simulink model "sedemo_rate_based_proc"  (Simulink 7.5)
settings: Solver=VariableStepDiscrete  StartTime=0.0  StopTime=86  MaxStep=Inf  RelTol=1e-3
undefined symbols (not defined in the file or in its folder): des_subsystemblock, des_subsysteminport, des_subsystemoutport, des_subsystemsupportblock
libraries: simeventstiming1 x7, simeventstranslate1 x7, simeventssink1 x5, simeventsattributes2 x5, simeventsgenerators1 x4, simeventsgates1 x3, simeventsrouting1 x3, simeventsserver1 x3, simeventsqueue1 x1, simeventsinfo x1
settings Model: Creator=The MathWorks Inc.
settings SolverCC: InsertRTBMode=Auto
settings OptimizationCC: InitFltsAndDblsToZero=on
settings DebuggingCC: SolverPrmCheckMsg=none  StrictBusMsg=Warning
settings SimEventsCC: propMaxDesBlkSimulEvents=10000  propDiagAttribOutput=0  propDiagFcnCallOutput=0  propDiagStatOutput=0  propDiagChangeAttrib=0  propRNGIdenticalSeeds=0

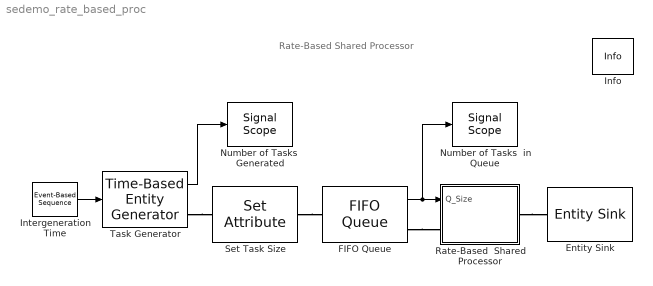
== system sedemo_rate_based_proc ==
  note: Rate-Based Shared Processor
  Entity Sink : simeventssink1/Entity Sink  Priority=1  SystemSampleTime=-1  AvailableForArrivals=on  StatNumberArrived=Off
  FIFO Queue : simeventsqueue1/FIFO Queue  Priority=1  SystemSampleTime=-1  Capacity=10  EnableTOPort=off  StatNumberDeparted=Off  StatNumberInBlock=On  StatPendingEntity=Off  StatAverageWait=Off  StatAverageQueueLength=Off  StatNumberTimedout=Off
  Info : simeventsinfo/Info  SystemSampleTime=-1
  Intergeneration Time : simeventsgenerators1/Signal Generators/Event-Based Sequence  SystemSampleTime=-1  VectorOutputValues=rand(1,85)*2.4  FormOutputOpt=Cyclic repetition  IsProcessed=on  isConnected=1
  Number of Tasks  Generated : simeventssink1/Signal Scope  Priority=1  SystemSampleTime=-1  PlotType=Stair  InputType=Signal  NumInputs=1  AttributeNameY=Count  XInputOptionSignal=Event time  XInputOptionEntity=Event time  AttributeNameX=Count  EnableEntityOutport=on  XMin=0  XMax=100  XLimitExceededOption=Stretch axis limits  YLimitExceededOption=Stretch axis limits  AxisGrid=on  AxisLegend=off  LineDisables=""  LineColors=b  LineStyles=-  LineMarkers=None  OpenScopeAtSimStart=on  Title=Number of Tasks Generated  YLabel=Number of Tasks  XLabel=Time  FigurePosition=[116 516 360 184]  AxisZoom=off  DataStoreOption=Limited  DataPointsLimit=10000  StatNumberArrived=Off  ShowCountPlotted=off  ShowToolbar=off
      settings: YMin=0  YMax=100
  Number of Tasks  in Queue : simeventssink1/Signal Scope  Priority=1  SystemSampleTime=-1  PlotType=Stair  InputType=Signal  NumInputs=1  AttributeNameY=Count  XInputOptionSignal=Event time  XInputOptionEntity=Event time  AttributeNameX=Count  EnableEntityOutport=on  XMin=0  XMax=100  XLimitExceededOption=Stretch axis limits  YLimitExceededOption=Stretch axis limits  AxisGrid=on  AxisLegend=off  LineDisables=""  LineColors="1  0  1"  LineStyles=-  LineMarkers=None  OpenScopeAtSimStart=on  Title=Number of Tasks Waiting for Service  YLabel=Number of Tasks  XLabel=Time  FigurePosition=[483 516 360 184]  AxisZoom=off  DataStoreOption=Limited  DataPointsLimit=10000  StatNumberArrived=Off  ShowCountPlotted=off  ShowToolbar=off
      settings: YMin=0  YMax=4
  Rate-Based  Shared Processor : Subsystem
  Set Task Size : simeventsattributes2/Set Attribute  Priority=1  DialogController=des_ddg_create  DialogControllerArgs=DataTag62  SystemSampleTime=-1  AttributeFrom=Dialog  AttributeName=ResidualWork  AttributeTreatAsVector=1  AttributeValue=1  AttributeCreate=on  StatNumberDeparted=Off  EvaluatedAttributeValue={1}
  Task Generator : simeventsgenerators1/Entity Generators/Time-Based Entity Generator  Priority=1  DialogController=des_ddg_create  DialogControllerArgs=DataTag64  SystemSampleTime=-1  GenerateEntitiesUpon=Intergeneration time from port t  Distribution=Exponential  Minimum=0  Maximum=1  Mean=2  InitialSeed=9675678  Period=1  PriorityEntityGeneration=300  GenerateEntityAtSimulationStart=on  ResponseWhenBlocked=Pause generation  ResponseWhenUnblocked=Immediate restart  EntityType=Blank  StatNumberDeparted=On  StatPendingEntity=Off  StatAverageIntergenerationTime=Off
  wires:
  FIFO Queue/1 -> Rate-Based  Shared Processor/1(Q_Size), Number of Tasks  in Queue/1
  Intergeneration Time/1 -> Task Generator/1
  Task Generator/1 -> Number of Tasks  Generated/1
  connections:
  Task Generator/RConn1 -- Set Task Size/LConn1
  FIFO Queue/RConn1 -- Rate-Based  Shared Processor/LConn1
  Rate-Based  Shared Processor/RConn1 -- Entity Sink/LConn1
  Set Task Size/RConn1 -- FIFO Queue/LConn1

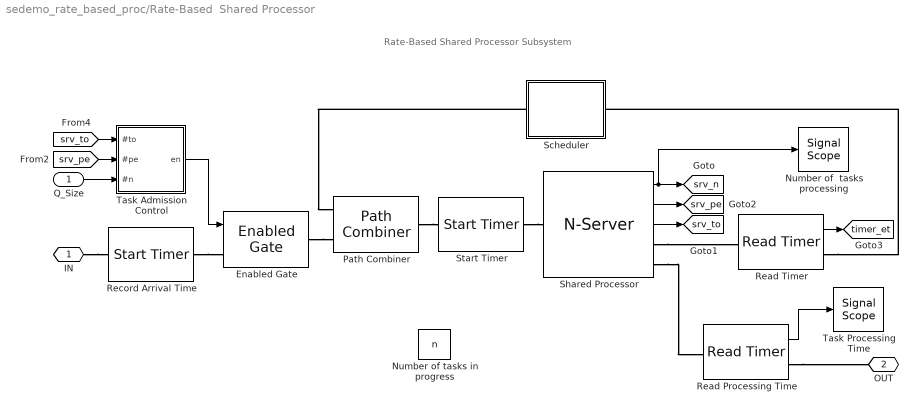
== system sedemo_rate_based_proc/Rate-Based  Shared Processor ==
  note: Rate-Based Shared Processor Subsystem
  Q_Size : Inport  OutDataType=sfix(16)  OutScaling=2^0
  Enabled Gate : simeventsgates1/Enabled Gate  Priority=1  SystemSampleTime=-1  SpecifyEventPriority=off  PriorityGateEnableOpenClose=2000  StatNumberDeparted=Off
  Number of  tasks processing : simeventssink1/Signal Scope  Priority=1  SystemSampleTime=-1  PlotType=Stair  InputType=Signal  NumInputs=1  AttributeNameY=Count  XInputOptionSignal=Event time  XInputOptionEntity=Event time  AttributeNameX=Count  EnableEntityOutport=on  XMin=0  XMax=100  XLimitExceededOption=Stretch axis limits  YLimitExceededOption=Stretch axis limits  AxisGrid=on  AxisLegend=off  LineDisables=""  LineColors="1  0  0"  LineStyles=-  LineMarkers=None  OpenScopeAtSimStart=on  Title=Number of Tasks Being Processed  YLabel=Number of Tasks  XLabel=Time  FigurePosition=[116 283 360 185]  AxisZoom=off  DataStoreOption=Limited  DataPointsLimit=10000  StatNumberArrived=Off  ShowCountPlotted=off  ShowToolbar=off
      settings: YMin=0  YMax=6
  Number of tasks in progress : DataStoreMemory  DataStoreName=n  OutDataType=sfix(16)  OutScaling=2^0
  Path Combiner : simeventsrouting1/Path Combiner  Priority=1  SystemSampleTime=-1  NumberInputPorts=2  InputPortPrecedence=IN1 port  InitialSeed=45675  SpecifyEventPriority=off  PriorityPathCombinerPortPrecedenceSelection=4100  StatNumberDeparted=Off  StatLastArrivalPort=Off  EvaluatedNumPorts=2
  Read Processing Time : simeventstiming1/Read Timer  Priority=0  SystemSampleTime=-1  TimerTag=ProcessingTime  TimerModeOption=Error  TimerStop=off  StatNumberDeparted=Off  StatTimerNumberDeparted=Off  StatTimeElapsed=On  StatAverageTimeElapsed=Off
  Read Timer : simeventstiming1/Read Timer  Priority=0  SystemSampleTime=-1  TimerTag=ServiceTime  TimerModeOption=Error  TimerStop=off  StatNumberDeparted=Off  StatTimerNumberDeparted=Off  StatTimeElapsed=On  StatAverageTimeElapsed=Off
  Record Arrival Time : simeventstiming1/Start Timer  Priority=0  SystemSampleTime=-1  TimerTag=ProcessingTime  TimerStartedOption=Warn and continue  StatNumberDeparted=Off
  Scheduler : Subsystem
  Shared Processor : simeventsserver1/N-Server  Priority=1  SystemSampleTime=-1  NumberOfServers=5  ServiceTimeFrom=Dialog  ServiceTime=0  AttributeName=ServiceTime  PriorityServiceCompletion=700  EnableTOPort=on  StatNumberDeparted=Off  StatNumberInBlock=On  StatPendingEntity=Off  StatNumberPending=On  StatAverageWait=Off  StatUtilization=Off  StatNumberTimedout=On
  Start Timer : simeventstiming1/Start Timer  Priority=0  SystemSampleTime=-1  TimerTag=ServiceTime  TimerStartedOption=Restart  StatNumberDeparted=Off
  Task Admission Control : Subsystem  LoadFcn=des_subsystemblock(gcb, 'load');  InitFcn=des_subsystemblock(gcb, 'init');  StartFcn=des_subsystemblock(gcb, 'start');  StopFcn=des_subsystemblock(gcb, 'stop');
      settings: CopyFcn=des_subsystemblock(gcb, 'copy');  DeleteFcn=des_subsystemblock(gcb, 'delete');  UndoDeleteFcn=des_subsystemblock(gcb, 'undodelete');  ModelCloseFcn=des_subsystemblock(gcb, 'modelclose');  PreSaveFcn=des_subsystemblock(gcb, 'presave');  NameChangeFcn=des_subsystemblock(gcb, 'namechange');  ParentCloseFcn=des_subsystemblock(gcb, 'parentclose');  ErrorFcn=des_subsystemerror
  Task Processing Time : simeventssink1/Signal Scope  Priority=1  SystemSampleTime=-1  PlotType=Stem  InputType=Signal  NumInputs=1  AttributeNameY=Count  XInputOptionSignal=Event time  XInputOptionEntity=Event time  AttributeNameX=Count  EnableEntityOutport=on  XMin=0  XMax=100  XLimitExceededOption=Stretch axis limits  YLimitExceededOption=Stretch axis limits  AxisGrid=on  AxisLegend=off  LineDisables=""  LineColors="0  0  1"  LineStyles=-  LineMarkers=diamond  OpenScopeAtSimStart=on  Title=Task Processing Time  YLabel=Processing Time  XLabel=Departure Time  FigurePosition=[483 283 360 185]  AxisZoom=off  DataStoreOption=Limited  DataPointsLimit=10000  StatNumberArrived=Off  ShowCountPlotted=off  ShowToolbar=off
      settings: YMin=0  YMax=6
  IN : PMIOPort  Port=1  Side=Left
  OUT : PMIOPort  Port=2  Side=Right
  tag scope: srv_n=global, srv_pe=global, srv_to=global, timer_et=global
  wires:
  Read Timer/1 -> [timer_et]
  Shared Processor/1 -> [srv_n], Number of  tasks processing/1
  Shared Processor/2 -> [srv_pe]
  Shared Processor/3 -> [srv_to]
  Task Admission Control/1(en) -> Enabled Gate/1
  Q_Size/1 -> Task Admission Control/3(#n)
  [srv_pe] -> Task Admission Control/2(#pe)
  [srv_to] -> Task Admission Control/1(#to)
  Read Processing Time/1 -> Task Processing Time/1
  connections:
  Start Timer/RConn1 -- Shared Processor/LConn1
  Shared Processor/RConn1 -- Read Timer/LConn1
  Path Combiner/RConn1 -- Start Timer/LConn1
  Enabled Gate/RConn1 -- Path Combiner/LConn2
  Read Timer/RConn1 -- Scheduler/LConn1
  Scheduler/RConn1 -- Path Combiner/LConn1
  Record Arrival Time/RConn1 -- Enabled Gate/LConn1
  IN/RConn1 -- Record Arrival Time/LConn1
  Shared Processor/RConn2 -- Read Processing Time/LConn1
  Read Processing Time/RConn1 -- OUT/RConn1

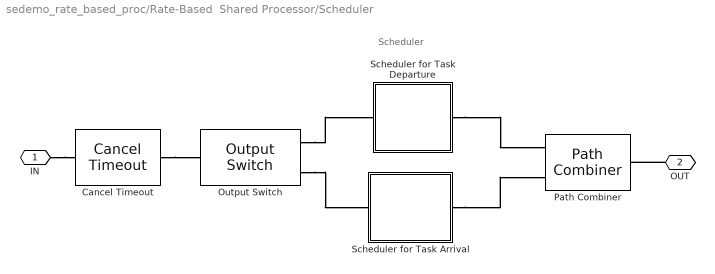
== system sedemo_rate_based_proc/Rate-Based  Shared Processor/Scheduler ==
  note: Scheduler
  Cancel Timeout : simeventstiming1/Cancel Timeout  Priority=0  SystemSampleTime=-1  TimeoutTag=ResidualServiceTime  TimeoutModeOption=Continue  TimeoutCancelledOption=Continue  StatNumberDeparted=Off  StatTimeoutNumberDeparted=Off  StatResidualTimeout=Off  StatAverageResidualTimeout=Off
  Output Switch : simeventsrouting1/Output Switch  Priority=1  SystemSampleTime=-1  NumberOutputPorts=2  SwitchingCriterion=First port that is not blocked  InitialSeed=34567  AttributeName=Attribute1  InitialConditionsOpt=off  InitialConditions=1  EntityBufferOpt=off  SpecifyEventPriority=off  PriorityOutputSwitchSelectPort=4100  TimeoutPortOpt=off  StatNumberDeparted=Off  StatNumberTimedOut=Off  StatPendingEntity=Off  StatLastDeparturePort=Off  EvaluatedNumPorts=2
  Path Combiner : simeventsrouting1/Path Combiner  Priority=1  SystemSampleTime=-1  NumberInputPorts=2  InputPortPrecedence=IN1 port  InitialSeed=45675  SpecifyEventPriority=off  PriorityPathCombinerPortPrecedenceSelection=4100  StatNumberDeparted=Off  StatLastArrivalPort=Off  EvaluatedNumPorts=2
  Scheduler for Task Arrival : Subsystem
  Scheduler for Task Departure : Subsystem
  IN : PMIOPort  Port=1  Side=Left
  OUT : PMIOPort  Port=2  Side=Right
  connections:
  Cancel Timeout/RConn1 -- Output Switch/LConn1
  Output Switch/RConn1 -- Scheduler for Task Departure/LConn1
  Output Switch/RConn2 -- Scheduler for Task Arrival/LConn1
  Scheduler for Task Departure/RConn1 -- Path Combiner/LConn1
  Scheduler for Task Arrival/RConn1 -- Path Combiner/LConn2
  IN/RConn1 -- Cancel Timeout/LConn1
  OUT/RConn1 -- Path Combiner/RConn1

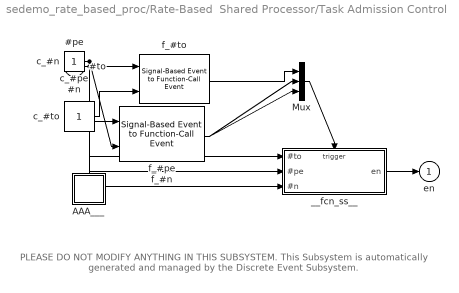
== system sedemo_rate_based_proc/Rate-Based  Shared Processor/Task Admission Control ==
  note: PLEASE DO NOT MODIFY ANYTHING IN THIS SUBSYSTEM.
      | This Subsystem is automatically generated and
      | managed by the Discrete Event Subsystem.
  #to : Inport  DataType=double  OutDataType=sfix(16)  OutScaling=2^0  OutDataTypeStr=double
  #pe : Inport  Port=2  DataType=double  OutDataType=sfix(16)  OutScaling=2^0  OutDataTypeStr=double
  #n : Inport  Port=3  DataType=double  OutDataType=sfix(16)  OutScaling=2^0  OutDataTypeStr=double
  AAA___ : Subsystem  LoadFcn=des_subsystemsupportblock(gcb, 'load');  InitFcn=des_subsystemsupportblock(gcb, 'init');  StartFcn=des_subsystemsupportblock(gcb, 'start');  StopFcn=des_subsystemsupportblock(gcb, 'stop');
      settings: CopyFcn=des_subsystemsupportblock(gcb, 'copy');  DeleteFcn=des_subsystemsupportblock(gcb, 'delete');  UndoDeleteFcn=des_subsystemsupportblock(gcb, 'undodelete');  ModelCloseFcn=des_subsystemsupportblock(gcb, 'modelclose');  PreSaveFcn=des_subsystemsupportblock(gcb, 'presave');  NameChangeFcn=des_subsystemsupportblock(gcb, 'namechange');  OpenFcn=des_subsystemsupportblock(gcb, 'open');  ParentCloseFcn=des_subsystemsupportblock(gcb, 'parentclose');
  Mux : Mux  Inputs=3
  __fcn_ss__ : Subsystem  TreatAsAtomicUnit=on
      settings: PropExecContextOutsideSubsystem=on
  c_#n : Constant  OutDataType=sfix(16)  OutScaling=2^0
  c_#pe : Constant  OutDataType=sfix(16)  OutScaling=2^0
  c_#to : Constant  OutDataType=sfix(16)  OutScaling=2^0
  f_#n : simeventstranslate1/Signal-Based Event to Function-Call Event  Priority=1  SystemSampleTime=-1  GenerateFunctionCallUpon=Change in signal from port vc  SignalEdgeOption=Rising  EnableE1Port=on  EnableF2Port=off  EnableE2Port=off  SpecifyEventPriority=off  PriorityFunctionCall=600  FunctionCallDelayFrom=Dialog  DelayFunctionCall=0  StatNumberF1Calls=Off  StatNumberF2Calls=Off  MaskBlockType=DESS_EVENT_PORT
  f_#pe : simeventstranslate1/Signal-Based Event to Function-Call Event  Priority=1  SystemSampleTime=-1  GenerateFunctionCallUpon=Change in signal from port vc  SignalEdgeOption=Rising  EnableE1Port=on  EnableF2Port=off  EnableE2Port=off  SpecifyEventPriority=off  PriorityFunctionCall=800  FunctionCallDelayFrom=Dialog  DelayFunctionCall=0  StatNumberF1Calls=Off  StatNumberF2Calls=Off  MaskBlockType=DESS_EVENT_PORT
  f_#to : simeventstranslate1/Signal-Based Event to Function-Call Event  Priority=1  SystemSampleTime=-1  GenerateFunctionCallUpon=Change in signal from port vc  SignalEdgeOption=Rising  EnableE1Port=on  EnableF2Port=off  EnableE2Port=off  SpecifyEventPriority=off  PriorityFunctionCall=500  FunctionCallDelayFrom=Dialog  DelayFunctionCall=0  StatNumberF1Calls=Off  StatNumberF2Calls=Off  MaskBlockType=DESS_EVENT_PORT
  en : Outport  OutDataType=sfix(16)  OutScaling=2^0
  wires:
  c_#pe/1 -> f_#pe/2
  f_#pe/1 -> Mux/2
  Mux/1 -> __fcn_ss__/Trigger
  c_#to/1 -> f_#to/2
  f_#to/1 -> Mux/1
  __fcn_ss__/1(en) -> en/1
  f_#n/1 -> Mux/3
  c_#n/1 -> f_#n/2
  #to/1 -> f_#to/1, __fcn_ss__/1(#to)
  #pe/1 -> f_#pe/1, __fcn_ss__/2(#pe)
  #n/1 -> f_#n/1, __fcn_ss__/3(#n)

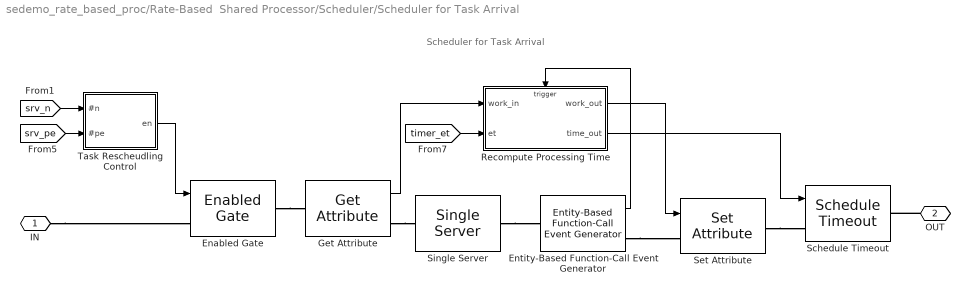
== system sedemo_rate_based_proc/Rate-Based  Shared Processor/Scheduler/Scheduler for Task Arrival ==
  note: Scheduler for Task Arrival
  Enabled Gate : simeventsgates1/Enabled Gate  Priority=1  SystemSampleTime=-1  SpecifyEventPriority=off  PriorityGateEnableOpenClose=2000  StatNumberDeparted=Off
  Entity-Based Function-Call Event Generator : simeventsgenerators1/Event Generators/Entity-Based Function-Call Event Generator  Priority=1  SystemSampleTime=-1  TimingFunctionCallF1=Before entity departure  EnableE1Port=off  EnableF2Port=off  TimingFunctionCallF2=After entity departure  EnableE2Port=off  StatNumberDeparted=Off  StatNumberF1Calls=Off  StatNumberF2Calls=Off  IsInsideAFB=off
  Get Attribute : simeventsattributes2/Get Attribute  Priority=1  DialogController=des_ddg_create  DialogControllerArgs=DataTag16  SystemSampleTime=-1  AttributeName=ResidualWork  AttributeMissing=Error  AttributeDefaultValue=1  AttributeSendTiming=After entity departure  AttributeTreatAsVector=1  StatNumberDeparted=Off  EvaluatedDefaultAttributeValue={[]}
  Recompute Processing Time : Subsystem  TreatAsAtomicUnit=on
      settings: PropExecContextOutsideSubsystem=on
  Schedule Timeout : simeventstiming1/Schedule Timeout  Priority=0  SystemSampleTime=-1  TimeoutTag=ResidualServiceTime  TimeoutIntervalFrom=Signal port ti  TimeoutInterval=1  AttributeName=TimeoutAttribute  PriorityTimeout=1700  TimeoutScheduledOption=Error  TimeoutNoDestination=Error  StatNumberDeparted=Off
  Set Attribute : simeventsattributes2/Set Attribute  Priority=1  DialogController=des_ddg_create  DialogControllerArgs=DataTag19  SystemSampleTime=-1  AttributeFrom=Signal port  AttributeName=ResidualWork  AttributeTreatAsVector=1  AttributeValue=1  AttributeCreate=on  StatNumberDeparted=Off  EvaluatedAttributeValue={[]}
  Single Server : simeventsserver1/Single Server  Priority=1  SystemSampleTime=-1  ServiceTimeFrom=Dialog  ServiceTime=0  AttributeName=ServiceTime  PriorityServiceCompletion=50  PermitPreemption=off  SortingAttributeName=PriorityAttributeName  SortingDirection=Ascending  WriteToAttribute=off  ResidualAttributeName=ResidualServiceTime  CreateAttribute=on  EnableTOPort=off  StatNumberDeparted=Off  StatNumberInBlock=Off  StatNumberPreempted=Off  StatPendingEntity=Off  StatAverageWait=Off  StatUtilization=Off  StatNumberTimedout=Off
  Task Rescheudling Control : Subsystem  LoadFcn=des_subsystemblock(gcb, 'load');  InitFcn=des_subsystemblock(gcb, 'init');  StartFcn=des_subsystemblock(gcb, 'start');  StopFcn=des_subsystemblock(gcb, 'stop');
      settings: CopyFcn=des_subsystemblock(gcb, 'copy');  DeleteFcn=des_subsystemblock(gcb, 'delete');  UndoDeleteFcn=des_subsystemblock(gcb, 'undodelete');  ModelCloseFcn=des_subsystemblock(gcb, 'modelclose');  PreSaveFcn=des_subsystemblock(gcb, 'presave');  NameChangeFcn=des_subsystemblock(gcb, 'namechange');  ParentCloseFcn=des_subsystemblock(gcb, 'parentclose');  ErrorFcn=des_subsystemerror
  IN : PMIOPort  Port=1  Side=Left
  OUT : PMIOPort  Port=2  Side=Right
  wires:
  Get Attribute/1 -> Recompute Processing Time/1(work_in)
  Recompute Processing Time/1(work_out) -> Set Attribute/1
  Recompute Processing Time/2(time_out) -> Schedule Timeout/1
  [srv_n] -> Task Rescheudling Control/1(#n)
  [srv_pe] -> Task Rescheudling Control/2(#pe)
  [timer_et] -> Recompute Processing Time/2(et)
  Task Rescheudling Control/1(en) -> Enabled Gate/1
  Entity-Based Function-Call Event Generator/1 -> Recompute Processing Time/Trigger
  connections:
  Enabled Gate/RConn1 -- Get Attribute/LConn1
  Get Attribute/RConn1 -- Single Server/LConn1
  Set Attribute/RConn1 -- Schedule Timeout/LConn1
  OUT/RConn1 -- Schedule Timeout/RConn1
  IN/RConn1 -- Enabled Gate/LConn1
  Entity-Based Function-Call Event Generator/RConn1 -- Set Attribute/LConn1
  Single Server/RConn1 -- Entity-Based Function-Call Event Generator/LConn1

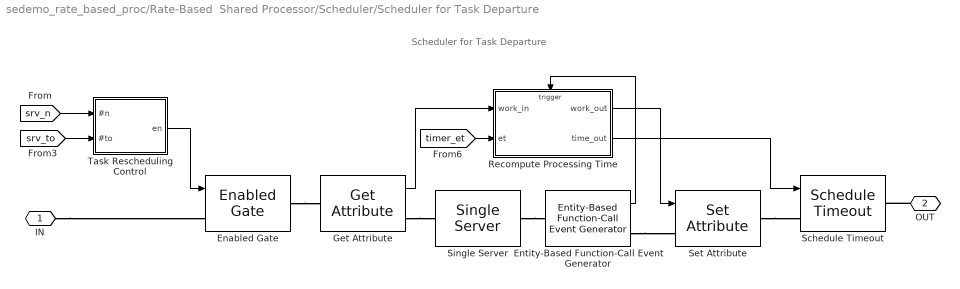
== system sedemo_rate_based_proc/Rate-Based  Shared Processor/Scheduler/Scheduler for Task Departure ==
  note: Scheduler for Task Departure
  Enabled Gate : simeventsgates1/Enabled Gate  Priority=1  SystemSampleTime=-1  SpecifyEventPriority=off  PriorityGateEnableOpenClose=2000  StatNumberDeparted=Off
  Entity-Based Function-Call Event Generator : simeventsgenerators1/Event Generators/Entity-Based Function-Call Event Generator  Priority=1  SystemSampleTime=-1  TimingFunctionCallF1=Before entity departure  EnableE1Port=off  EnableF2Port=off  TimingFunctionCallF2=After entity departure  EnableE2Port=off  StatNumberDeparted=Off  StatNumberF1Calls=Off  StatNumberF2Calls=Off  IsInsideAFB=off
  Get Attribute : simeventsattributes2/Get Attribute  Priority=1  DialogController=des_ddg_create  DialogControllerArgs=DataTag33  SystemSampleTime=-1  AttributeName=ResidualWork  AttributeMissing=Error  AttributeDefaultValue=1  AttributeSendTiming=After entity departure  AttributeTreatAsVector=1  StatNumberDeparted=Off  EvaluatedDefaultAttributeValue={[]}
  Recompute Processing Time : Subsystem  TreatAsAtomicUnit=on
      settings: PropExecContextOutsideSubsystem=on
  Schedule Timeout : simeventstiming1/Schedule Timeout  Priority=0  SystemSampleTime=-1  TimeoutTag=ResidualServiceTime  TimeoutIntervalFrom=Signal port ti  TimeoutInterval=1  AttributeName=TimeoutAttribute  PriorityTimeout=1700  TimeoutScheduledOption=Error  TimeoutNoDestination=Error  StatNumberDeparted=Off
  Set Attribute : simeventsattributes2/Set Attribute  Priority=1  DialogController=des_ddg_create  DialogControllerArgs=DataTag36  SystemSampleTime=-1  AttributeFrom=Signal port  AttributeName=ResidualWork  AttributeTreatAsVector=1  AttributeValue=1  AttributeCreate=on  StatNumberDeparted=Off  EvaluatedAttributeValue={[]}
  Single Server : simeventsserver1/Single Server  Priority=1  SystemSampleTime=-1  ServiceTimeFrom=Dialog  ServiceTime=0  AttributeName=ServiceTime  PriorityServiceCompletion=50  PermitPreemption=off  SortingAttributeName=PriorityAttributeName  SortingDirection=Ascending  WriteToAttribute=off  ResidualAttributeName=ResidualServiceTime  CreateAttribute=on  EnableTOPort=off  StatNumberDeparted=Off  StatNumberInBlock=Off  StatNumberPreempted=Off  StatPendingEntity=Off  StatAverageWait=Off  StatUtilization=Off  StatNumberTimedout=Off
  Task Rescheduling Control : Subsystem  LoadFcn=des_subsystemblock(gcb, 'load');  InitFcn=des_subsystemblock(gcb, 'init');  StartFcn=des_subsystemblock(gcb, 'start');  StopFcn=des_subsystemblock(gcb, 'stop');
      settings: CopyFcn=des_subsystemblock(gcb, 'copy');  DeleteFcn=des_subsystemblock(gcb, 'delete');  UndoDeleteFcn=des_subsystemblock(gcb, 'undodelete');  ModelCloseFcn=des_subsystemblock(gcb, 'modelclose');  PreSaveFcn=des_subsystemblock(gcb, 'presave');  NameChangeFcn=des_subsystemblock(gcb, 'namechange');  ParentCloseFcn=des_subsystemblock(gcb, 'parentclose');  ErrorFcn=des_subsystemerror
  IN : PMIOPort  Port=1  Side=Left
  OUT : PMIOPort  Port=2  Side=Right
  wires:
  Task Rescheduling Control/1(en) -> Enabled Gate/1
  Get Attribute/1 -> Recompute Processing Time/1(work_in)
  Recompute Processing Time/2(time_out) -> Schedule Timeout/1
  Recompute Processing Time/1(work_out) -> Set Attribute/1
  [srv_n] -> Task Rescheduling Control/1(#n)
  [srv_to] -> Task Rescheduling Control/2(#to)
  [timer_et] -> Recompute Processing Time/2(et)
  Entity-Based Function-Call Event Generator/1 -> Recompute Processing Time/Trigger
  connections:
  Enabled Gate/RConn1 -- Get Attribute/LConn1
  Set Attribute/RConn1 -- Schedule Timeout/LConn1
  OUT/RConn1 -- Schedule Timeout/RConn1
  IN/RConn1 -- Enabled Gate/LConn1
  Get Attribute/RConn1 -- Single Server/LConn1
  Single Server/RConn1 -- Entity-Based Function-Call Event Generator/LConn1
  Entity-Based Function-Call Event Generator/RConn1 -- Set Attribute/LConn1

== system sedemo_rate_based_proc/Rate-Based  Shared Processor/Task Admission Control/AAA___ ==

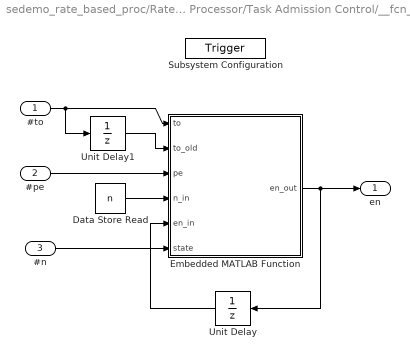
== system sedemo_rate_based_proc/Rate-Based  Shared Processor/Task Admission Control/__fcn_ss__ ==
  #to : Inport  LoadFcn=des_subsysteminport(gcb, 'load');  InitFcn=des_subsysteminport(gcb, 'init');  StartFcn=des_subsysteminport(gcb, 'start');  StopFcn=des_subsysteminport(gcb, 'stop');  OutDataType=sfix(16)  OutScaling=2^0  mask(Discrete Event Inport){PermitSubsystemEvents=on, TypeOfEvent=Change in signal, SignalEdgeOption=Rising, SpecifyEventPriority=off, PrioritySubsystemEvent=500}
      mask prompts: PermitSubsystemEvents "Execute subsystem upon signal-based events"; TypeOfEvent "Type of signal-based event:"; SignalEdgeOption "Type of change in signal value:"; SpecifyEventPriority "Resolve simultaneous signal updates according to event priority"; PrioritySubsystemEvent "Event priority:"
      mask help: Input port for a Discrete Event Subsystem block. This block can conditionally execute the subsystem upon signal-based events that meet specified criteria.
      mask init:
      | des_subsystemmask(gcb, 'init','apply')
      settings: CopyFcn=des_subsysteminport(gcb, 'copy');  DeleteFcn=des_subsysteminport(gcb, 'delete');  UndoDeleteFcn=des_subsysteminport(gcb, 'undodelete');  ModelCloseFcn=des_subsysteminport(gcb, 'modelclose');  PreSaveFcn=des_subsysteminport(gcb, 'presave');  NameChangeFcn=des_subsysteminport(gcb, 'namechange');  ParentCloseFcn=des_subsysteminport(gcb, 'parentclose');
      mask Help: helpview(simeventsbhelp);
      mask StyleString: checkbox,popup(Change in signal|Trigger|Sample time hit),popup(Rising|Falling|Either),checkbox,edit
      mask CallbackString: des_subsystemmask(gcb, 'cbPermitSubsystemEvents', 'noapply');|des_subsystemmask(gcb,'cbTypeOfEvent','noapply');||des_subsystemmask(gcb, 'cbSpecifyEventPriority', 'noapply');|
  #pe : Inport  LoadFcn=des_subsysteminport(gcb, 'load');  InitFcn=des_subsysteminport(gcb, 'init');  StartFcn=des_subsysteminport(gcb, 'start');  StopFcn=des_subsysteminport(gcb, 'stop');  Port=2  OutDataType=sfix(16)  OutScaling=2^0  mask(Discrete Event Inport){PermitSubsystemEvents=on, TypeOfEvent=Change in signal, SignalEdgeOption=Rising, SpecifyEventPriority=off, PrioritySubsystemEvent=800}
      mask prompts: PermitSubsystemEvents "Execute subsystem upon signal-based events"; TypeOfEvent "Type of signal-based event:"; SignalEdgeOption "Type of change in signal value:"; SpecifyEventPriority "Resolve simultaneous signal updates according to event priority"; PrioritySubsystemEvent "Event priority:"
      mask help: Input port for a Discrete Event Subsystem block. This block can conditionally execute the subsystem upon signal-based events that meet specified criteria.
      mask init:
      | des_subsystemmask(gcb, 'init','apply')
      settings: CopyFcn=des_subsysteminport(gcb, 'copy');  DeleteFcn=des_subsysteminport(gcb, 'delete');  UndoDeleteFcn=des_subsysteminport(gcb, 'undodelete');  ModelCloseFcn=des_subsysteminport(gcb, 'modelclose');  PreSaveFcn=des_subsysteminport(gcb, 'presave');  NameChangeFcn=des_subsysteminport(gcb, 'namechange');  ParentCloseFcn=des_subsysteminport(gcb, 'parentclose');
      mask Help: helpview(simeventsbhelp);
      mask StyleString: checkbox,popup(Change in signal|Trigger|Sample time hit),popup(Rising|Falling|Either),checkbox,edit
      mask CallbackString: des_subsystemmask(gcb, 'cbPermitSubsystemEvents', 'noapply');|des_subsystemmask(gcb,'cbTypeOfEvent','noapply');||des_subsystemmask(gcb, 'cbSpecifyEventPriority', 'noapply');|
  #n : Inport  LoadFcn=des_subsysteminport(gcb, 'load');  InitFcn=des_subsysteminport(gcb, 'init');  StartFcn=des_subsysteminport(gcb, 'start');  StopFcn=des_subsysteminport(gcb, 'stop');  Port=3  OutDataType=sfix(16)  OutScaling=2^0  mask(Discrete Event Inport){PermitSubsystemEvents=on, TypeOfEvent=Change in signal, SignalEdgeOption=Rising, SpecifyEventPriority=off, PrioritySubsystemEvent=600}
      mask prompts: PermitSubsystemEvents "Execute subsystem upon signal-based events"; TypeOfEvent "Type of signal-based event:"; SignalEdgeOption "Type of change in signal value:"; SpecifyEventPriority "Resolve simultaneous signal updates according to event priority"; PrioritySubsystemEvent "Event priority:"
      mask help: Input port for a Discrete Event Subsystem block. This block can conditionally execute the subsystem upon signal-based events that meet specified criteria.
      mask init:
      | des_subsystemmask(gcb, 'init','apply')
      settings: CopyFcn=des_subsysteminport(gcb, 'copy');  DeleteFcn=des_subsysteminport(gcb, 'delete');  UndoDeleteFcn=des_subsysteminport(gcb, 'undodelete');  ModelCloseFcn=des_subsysteminport(gcb, 'modelclose');  PreSaveFcn=des_subsysteminport(gcb, 'presave');  NameChangeFcn=des_subsysteminport(gcb, 'namechange');  ParentCloseFcn=des_subsysteminport(gcb, 'parentclose');
      mask Help: helpview(simeventsbhelp);
      mask StyleString: checkbox,popup(Change in signal|Trigger|Sample time hit),popup(Rising|Falling|Either),checkbox,edit
      mask CallbackString: des_subsystemmask(gcb, 'cbPermitSubsystemEvents', 'noapply');|des_subsystemmask(gcb,'cbTypeOfEvent','noapply');||des_subsystemmask(gcb, 'cbSpecifyEventPriority', 'noapply');|
  Subsystem Configuration : TriggerPort  TriggerType=function-call
      settings: CopyFcn=des_subsystemconfigblock(gcb, 'copy');  DeleteFcn=des_subsystemconfigblock(gcb, 'delete');  UndoDeleteFcn=des_subsystemconfigblock(gcb, 'undodelete');
      mask Type: Subsystem Configuration
      mask Description: Configuration for a Discrete Event Subsystem block. Every discrete event subsystem window must contain exactly one copy of this configuration block. Do not delete this block.
      mask Help: helpview(simeventsbhelp);
      mask Display: disp('Do Not Delete');
  Data Store Read : DataStoreRead  DataStoreName=n  SampleTime=-1
  Embedded MATLAB Function : Stateflow chart  TreatAsAtomicUnit=on
  Unit Delay : UnitDelay  SampleTime=-1
  Unit Delay1 : UnitDelay  SampleTime=-1
  en : Outport  LoadFcn=des_subsystemoutport(gcb, 'load');  InitFcn=des_subsystemoutport(gcb, 'init');  StartFcn=des_subsystemoutport(gcb, 'start');  StopFcn=des_subsystemoutport(gcb, 'stop');  OutDataType=sfix(16)  OutScaling=2^0
      settings: CopyFcn=des_subsystemoutport(gcb, 'copy');  DeleteFcn=des_subsystemoutport(gcb, 'delete');  UndoDeleteFcn=des_subsystemoutport(gcb, 'undodelete');  ModelCloseFcn=des_subsystemoutport(gcb, 'modelclose');  PreSaveFcn=des_subsystemoutport(gcb, 'presave');  NameChangeFcn=des_subsystemoutport(gcb, 'namechange');  ParentCloseFcn=des_subsystemoutport(gcb, 'parentclose');
      mask Type: Discrete Event Outport
      mask Description: Provide an output port for a Discrete Event Subsystem block.
      mask Help: helpview(simeventsbhelp);
  wires:
  Unit Delay/1 -> Embedded MATLAB Function/5(en_in)
  Embedded MATLAB Function/1(en_out) -> Unit Delay/1, en/1
  Data Store Read/1 -> Embedded MATLAB Function/4(n_in)
  #to/1 -> Embedded MATLAB Function/1(to), Unit Delay1/1
  #pe/1 -> Embedded MATLAB Function/3(pe)
  Unit Delay1/1 -> Embedded MATLAB Function/2(to_old)
  #n/1 -> Embedded MATLAB Function/6(state)

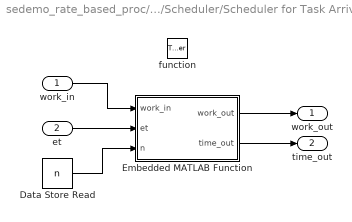
== system sedemo_rate_based_proc/Rate-Based  Shared Processor/Scheduler/Scheduler for Task Arrival/Recompute Processing Time ==
  work_in : Inport  OutDataType=sfix(16)  OutScaling=2^0
  et : Inport  Port=2  OutDataType=sfix(16)  OutScaling=2^0
  function : TriggerPort  TriggerType=function-call
  Data Store Read : DataStoreRead  DataStoreName=n  SampleTime=-1
  Embedded MATLAB Function : Stateflow chart  TreatAsAtomicUnit=on
  work_out : Outport  OutDataType=sfix(16)  OutScaling=2^0
  time_out : Outport  Port=2  OutDataType=sfix(16)  OutScaling=2^0
  wires:
  work_in/1 -> Embedded MATLAB Function/1(work_in)
  et/1 -> Embedded MATLAB Function/2(et)
  Data Store Read/1 -> Embedded MATLAB Function/3(n)
  Embedded MATLAB Function/1(work_out) -> work_out/1
  Embedded MATLAB Function/2(time_out) -> time_out/1

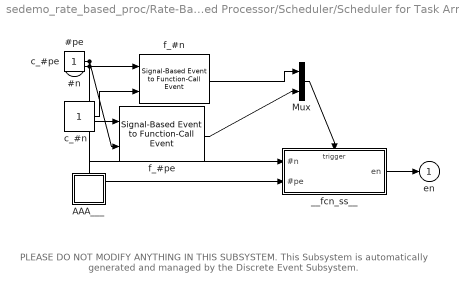
== system sedemo_rate_based_proc/Rate-Based  Shared Processor/Scheduler/Scheduler for Task Arrival/Task Rescheudling Control ==
  note: PLEASE DO NOT MODIFY ANYTHING IN THIS SUBSYSTEM.
      | This Subsystem is automatically generated and
      | managed by the Discrete Event Subsystem.
  #n : Inport  DataType=double  OutDataType=sfix(16)  OutScaling=2^0  OutDataTypeStr=double
  #pe : Inport  Port=2  DataType=double  OutDataType=sfix(16)  OutScaling=2^0  OutDataTypeStr=double
  AAA___ : Subsystem  LoadFcn=des_subsystemsupportblock(gcb, 'load');  InitFcn=des_subsystemsupportblock(gcb, 'init');  StartFcn=des_subsystemsupportblock(gcb, 'start');  StopFcn=des_subsystemsupportblock(gcb, 'stop');
      settings: CopyFcn=des_subsystemsupportblock(gcb, 'copy');  DeleteFcn=des_subsystemsupportblock(gcb, 'delete');  UndoDeleteFcn=des_subsystemsupportblock(gcb, 'undodelete');  ModelCloseFcn=des_subsystemsupportblock(gcb, 'modelclose');  PreSaveFcn=des_subsystemsupportblock(gcb, 'presave');  NameChangeFcn=des_subsystemsupportblock(gcb, 'namechange');  OpenFcn=des_subsystemsupportblock(gcb, 'open');  ParentCloseFcn=des_subsystemsupportblock(gcb, 'parentclose');
  Mux : Mux  Inputs=2
  __fcn_ss__ : Subsystem  TreatAsAtomicUnit=on
      settings: PropExecContextOutsideSubsystem=on
  c_#n : Constant  OutDataType=sfix(16)  OutScaling=2^0
  c_#pe : Constant  OutDataType=sfix(16)  OutScaling=2^0
  f_#n : simeventstranslate1/Signal-Based Event to Function-Call Event  Priority=1  SystemSampleTime=-1  GenerateFunctionCallUpon=Change in signal from port vc  SignalEdgeOption=Rising  EnableE1Port=on  EnableF2Port=off  EnableE2Port=off  SpecifyEventPriority=on  PriorityFunctionCall=600  FunctionCallDelayFrom=Dialog  DelayFunctionCall=0  StatNumberF1Calls=Off  StatNumberF2Calls=Off  MaskBlockType=DESS_EVENT_PORT
  f_#pe : simeventstranslate1/Signal-Based Event to Function-Call Event  Priority=1  SystemSampleTime=-1  GenerateFunctionCallUpon=Change in signal from port vc  SignalEdgeOption=Rising  EnableE1Port=on  EnableF2Port=off  EnableE2Port=off  SpecifyEventPriority=on  PriorityFunctionCall=600  FunctionCallDelayFrom=Dialog  DelayFunctionCall=0  StatNumberF1Calls=Off  StatNumberF2Calls=Off  MaskBlockType=DESS_EVENT_PORT
  en : Outport  OutDataType=sfix(16)  OutScaling=2^0
  wires:
  __fcn_ss__/1(en) -> en/1
  f_#n/1 -> Mux/1
  c_#n/1 -> f_#n/2
  Mux/1 -> __fcn_ss__/Trigger
  f_#pe/1 -> Mux/2
  c_#pe/1 -> f_#pe/2
  #n/1 -> f_#n/1, __fcn_ss__/1(#n)
  #pe/1 -> f_#pe/1, __fcn_ss__/2(#pe)

== system sedemo_rate_based_proc/Rate-Based  Shared Processor/Scheduler/Scheduler for Task Departure/Recompute Processing Time ==
  work_in : Inport  OutDataType=sfix(16)  OutScaling=2^0
  et : Inport  Port=2  OutDataType=sfix(16)  OutScaling=2^0
  function : TriggerPort  TriggerType=function-call
  Data Store Read : DataStoreRead  DataStoreName=n  SampleTime=-1
  Embedded MATLAB Function : Stateflow chart  TreatAsAtomicUnit=on
  work_out : Outport  OutDataType=sfix(16)  OutScaling=2^0
  time_out : Outport  Port=2  OutDataType=sfix(16)  OutScaling=2^0
  wires:
  work_in/1 -> Embedded MATLAB Function/1(work_in)
  et/1 -> Embedded MATLAB Function/2(et)
  Data Store Read/1 -> Embedded MATLAB Function/3(n)
  Embedded MATLAB Function/1(work_out) -> work_out/1
  Embedded MATLAB Function/2(time_out) -> time_out/1

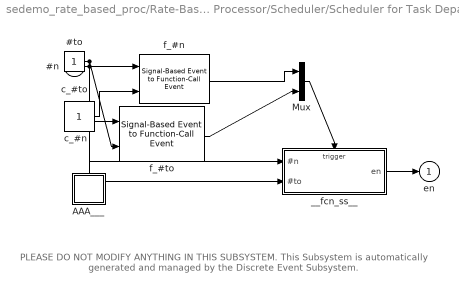
== system sedemo_rate_based_proc/Rate-Based  Shared Processor/Scheduler/Scheduler for Task Departure/Task Rescheduling Control ==
  note: PLEASE DO NOT MODIFY ANYTHING IN THIS SUBSYSTEM.
      | This Subsystem is automatically generated and
      | managed by the Discrete Event Subsystem.
  #n : Inport  DataType=double  OutDataType=sfix(16)  OutScaling=2^0  OutDataTypeStr=double
  #to : Inport  Port=2  DataType=double  OutDataType=sfix(16)  OutScaling=2^0  OutDataTypeStr=double
  AAA___ : Subsystem  LoadFcn=des_subsystemsupportblock(gcb, 'load');  InitFcn=des_subsystemsupportblock(gcb, 'init');  StartFcn=des_subsystemsupportblock(gcb, 'start');  StopFcn=des_subsystemsupportblock(gcb, 'stop');
      settings: CopyFcn=des_subsystemsupportblock(gcb, 'copy');  DeleteFcn=des_subsystemsupportblock(gcb, 'delete');  UndoDeleteFcn=des_subsystemsupportblock(gcb, 'undodelete');  ModelCloseFcn=des_subsystemsupportblock(gcb, 'modelclose');  PreSaveFcn=des_subsystemsupportblock(gcb, 'presave');  NameChangeFcn=des_subsystemsupportblock(gcb, 'namechange');  OpenFcn=des_subsystemsupportblock(gcb, 'open');  ParentCloseFcn=des_subsystemsupportblock(gcb, 'parentclose');
  Mux : Mux  Inputs=2
  __fcn_ss__ : Subsystem  TreatAsAtomicUnit=on
      settings: PropExecContextOutsideSubsystem=on
  c_#n : Constant  OutDataType=sfix(16)  OutScaling=2^0
  c_#to : Constant  OutDataType=sfix(16)  OutScaling=2^0
  f_#n : simeventstranslate1/Signal-Based Event to Function-Call Event  Priority=1  SystemSampleTime=-1  GenerateFunctionCallUpon=Change in signal from port vc  SignalEdgeOption=Rising  EnableE1Port=on  EnableF2Port=off  EnableE2Port=off  SpecifyEventPriority=on  PriorityFunctionCall=600  FunctionCallDelayFrom=Dialog  DelayFunctionCall=0  StatNumberF1Calls=Off  StatNumberF2Calls=Off  MaskBlockType=DESS_EVENT_PORT
  f_#to : simeventstranslate1/Signal-Based Event to Function-Call Event  Priority=1  SystemSampleTime=-1  GenerateFunctionCallUpon=Change in signal from port vc  SignalEdgeOption=Rising  EnableE1Port=on  EnableF2Port=off  EnableE2Port=off  SpecifyEventPriority=on  PriorityFunctionCall=600  FunctionCallDelayFrom=Dialog  DelayFunctionCall=0  StatNumberF1Calls=Off  StatNumberF2Calls=Off  MaskBlockType=DESS_EVENT_PORT
  en : Outport  OutDataType=sfix(16)  OutScaling=2^0
  wires:
  c_#to/1 -> f_#to/2
  f_#to/1 -> Mux/2
  Mux/1 -> __fcn_ss__/Trigger
  c_#n/1 -> f_#n/2
  f_#n/1 -> Mux/1
  __fcn_ss__/1(en) -> en/1
  #n/1 -> f_#n/1, __fcn_ss__/1(#n)
  #to/1 -> f_#to/1, __fcn_ss__/2(#to)

== system sedemo_rate_based_proc/Rate-Based  Shared Processor/Scheduler/Scheduler for Task Arrival/Task Rescheudling Control/AAA___ ==

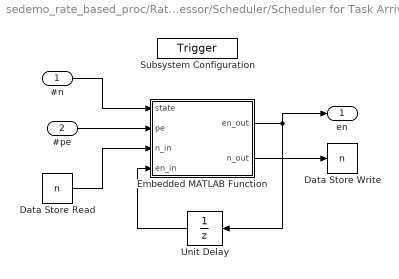
== system sedemo_rate_based_proc/Rate-Based  Shared Processor/Scheduler/Scheduler for Task Arrival/Task Rescheudling Control/__fcn_ss__ ==
  #n : Inport  LoadFcn=des_subsysteminport(gcb, 'load');  InitFcn=des_subsysteminport(gcb, 'init');  StartFcn=des_subsysteminport(gcb, 'start');  StopFcn=des_subsysteminport(gcb, 'stop');  OutDataType=sfix(16)  OutScaling=2^0  mask(Discrete Event Inport){PermitSubsystemEvents=on, TypeOfEvent=Change in signal, SignalEdgeOption=Rising, SpecifyEventPriority=on, PrioritySubsystemEvent=600}
      mask prompts: PermitSubsystemEvents "Execute subsystem upon signal-based events"; TypeOfEvent "Type of signal-based event:"; SignalEdgeOption "Type of change in signal value:"; SpecifyEventPriority "Resolve simultaneous signal updates according to event priority"; PrioritySubsystemEvent "Event priority:"
      mask help: Input port for a Discrete Event Subsystem block. This block can conditionally execute the subsystem upon signal-based events that meet specified criteria.
      mask init:
      | des_subsystemmask(gcb, 'init','apply')
      settings: CopyFcn=des_subsysteminport(gcb, 'copy');  DeleteFcn=des_subsysteminport(gcb, 'delete');  UndoDeleteFcn=des_subsysteminport(gcb, 'undodelete');  ModelCloseFcn=des_subsysteminport(gcb, 'modelclose');  PreSaveFcn=des_subsysteminport(gcb, 'presave');  NameChangeFcn=des_subsysteminport(gcb, 'namechange');  ParentCloseFcn=des_subsysteminport(gcb, 'parentclose');
      mask Help: helpview(simeventsbhelp);
      mask StyleString: checkbox,popup(Change in signal|Trigger|Sample time hit),popup(Rising|Falling|Either),checkbox,edit
      mask CallbackString: des_subsystemmask(gcb, 'cbPermitSubsystemEvents', 'noapply');|des_subsystemmask(gcb,'cbTypeOfEvent','noapply');||des_subsystemmask(gcb, 'cbSpecifyEventPriority', 'noapply');|
  #pe : Inport  LoadFcn=des_subsysteminport(gcb, 'load');  InitFcn=des_subsysteminport(gcb, 'init');  StartFcn=des_subsysteminport(gcb, 'start');  StopFcn=des_subsysteminport(gcb, 'stop');  Port=2  OutDataType=sfix(16)  OutScaling=2^0  mask(Discrete Event Inport){PermitSubsystemEvents=on, TypeOfEvent=Change in signal, SignalEdgeOption=Rising, SpecifyEventPriority=on, PrioritySubsystemEvent=600}
      mask prompts: PermitSubsystemEvents "Execute subsystem upon signal-based events"; TypeOfEvent "Type of signal-based event:"; SignalEdgeOption "Type of change in signal value:"; SpecifyEventPriority "Resolve simultaneous signal updates according to event priority"; PrioritySubsystemEvent "Event priority:"
      mask help: Input port for a Discrete Event Subsystem block. This block can conditionally execute the subsystem upon signal-based events that meet specified criteria.
      mask init:
      | des_subsystemmask(gcb, 'init','apply')
      settings: CopyFcn=des_subsysteminport(gcb, 'copy');  DeleteFcn=des_subsysteminport(gcb, 'delete');  UndoDeleteFcn=des_subsysteminport(gcb, 'undodelete');  ModelCloseFcn=des_subsysteminport(gcb, 'modelclose');  PreSaveFcn=des_subsysteminport(gcb, 'presave');  NameChangeFcn=des_subsysteminport(gcb, 'namechange');  ParentCloseFcn=des_subsysteminport(gcb, 'parentclose');
      mask Help: helpview(simeventsbhelp);
      mask StyleString: checkbox,popup(Change in signal|Trigger|Sample time hit),popup(Rising|Falling|Either),checkbox,edit
      mask CallbackString: des_subsystemmask(gcb, 'cbPermitSubsystemEvents', 'noapply');|des_subsystemmask(gcb,'cbTypeOfEvent','noapply');||des_subsystemmask(gcb, 'cbSpecifyEventPriority', 'noapply');|
  Subsystem Configuration : TriggerPort  TriggerType=function-call
      settings: CopyFcn=des_subsystemconfigblock(gcb, 'copy');  DeleteFcn=des_subsystemconfigblock(gcb, 'delete');  UndoDeleteFcn=des_subsystemconfigblock(gcb, 'undodelete');
      mask Type: Subsystem Configuration
      mask Description: Configuration for a Discrete Event Subsystem block. Every discrete event subsystem window must contain exactly one copy of this configuration block. Do not delete this block.
      mask Help: helpview(simeventsbhelp);
      mask Display: disp('Do Not Delete');
  Data Store Read : DataStoreRead  DataStoreName=n  SampleTime=-1
  Data Store Write : DataStoreWrite  DataStoreName=n  SampleTime=-1
  Embedded MATLAB Function : Stateflow chart  TreatAsAtomicUnit=on
  Unit Delay : UnitDelay  SampleTime=-1
  en : Outport  LoadFcn=des_subsystemoutport(gcb, 'load');  InitFcn=des_subsystemoutport(gcb, 'init');  StartFcn=des_subsystemoutport(gcb, 'start');  StopFcn=des_subsystemoutport(gcb, 'stop');  OutDataType=sfix(16)  OutScaling=2^0
      settings: CopyFcn=des_subsystemoutport(gcb, 'copy');  DeleteFcn=des_subsystemoutport(gcb, 'delete');  UndoDeleteFcn=des_subsystemoutport(gcb, 'undodelete');  ModelCloseFcn=des_subsystemoutport(gcb, 'modelclose');  PreSaveFcn=des_subsystemoutport(gcb, 'presave');  NameChangeFcn=des_subsystemoutport(gcb, 'namechange');  ParentCloseFcn=des_subsystemoutport(gcb, 'parentclose');
      mask Type: Discrete Event Outport
      mask Description: Provide an output port for a Discrete Event Subsystem block.
      mask Help: helpview(simeventsbhelp);
  wires:
  #pe/1 -> Embedded MATLAB Function/2(pe)
  #n/1 -> Embedded MATLAB Function/1(state)
  Data Store Read/1 -> Embedded MATLAB Function/3(n_in)
  Embedded MATLAB Function/2(n_out) -> Data Store Write/1
  Embedded MATLAB Function/1(en_out) -> en/1, Unit Delay/1
  Unit Delay/1 -> Embedded MATLAB Function/4(en_in)

== system sedemo_rate_based_proc/Rate-Based  Shared Processor/Scheduler/Scheduler for Task Departure/Task Rescheduling Control/AAA___ ==

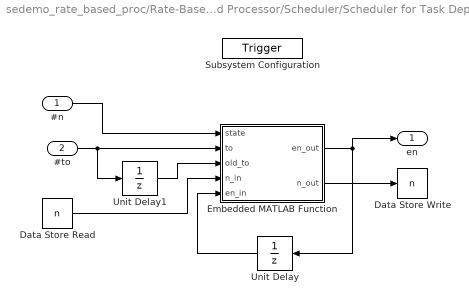
== system sedemo_rate_based_proc/Rate-Based  Shared Processor/Scheduler/Scheduler for Task Departure/Task Rescheduling Control/__fcn_ss__ ==
  #n : Inport  LoadFcn=des_subsysteminport(gcb, 'load');  InitFcn=des_subsysteminport(gcb, 'init');  StartFcn=des_subsysteminport(gcb, 'start');  StopFcn=des_subsysteminport(gcb, 'stop');  OutDataType=sfix(16)  OutScaling=2^0  mask(Discrete Event Inport){PermitSubsystemEvents=on, TypeOfEvent=Change in signal, SignalEdgeOption=Rising, SpecifyEventPriority=on, PrioritySubsystemEvent=600}
      mask prompts: PermitSubsystemEvents "Execute subsystem upon signal-based events"; TypeOfEvent "Type of signal-based event:"; SignalEdgeOption "Type of change in signal value:"; SpecifyEventPriority "Resolve simultaneous signal updates according to event priority"; PrioritySubsystemEvent "Event priority:"
      mask help: Input port for a Discrete Event Subsystem block. This block can conditionally execute the subsystem upon signal-based events that meet specified criteria.
      mask init:
      | des_subsystemmask(gcb, 'init','apply')
      settings: CopyFcn=des_subsysteminport(gcb, 'copy');  DeleteFcn=des_subsysteminport(gcb, 'delete');  UndoDeleteFcn=des_subsysteminport(gcb, 'undodelete');  ModelCloseFcn=des_subsysteminport(gcb, 'modelclose');  PreSaveFcn=des_subsysteminport(gcb, 'presave');  NameChangeFcn=des_subsysteminport(gcb, 'namechange');  ParentCloseFcn=des_subsysteminport(gcb, 'parentclose');
      mask Help: helpview(simeventsbhelp);
      mask StyleString: checkbox,popup(Change in signal|Trigger|Sample time hit),popup(Rising|Falling|Either),checkbox,edit
      mask CallbackString: des_subsystemmask(gcb, 'cbPermitSubsystemEvents', 'noapply');|des_subsystemmask(gcb,'cbTypeOfEvent','noapply');||des_subsystemmask(gcb, 'cbSpecifyEventPriority', 'noapply');|
  #to : Inport  LoadFcn=des_subsysteminport(gcb, 'load');  InitFcn=des_subsysteminport(gcb, 'init');  StartFcn=des_subsysteminport(gcb, 'start');  StopFcn=des_subsysteminport(gcb, 'stop');  Port=2  OutDataType=sfix(16)  OutScaling=2^0  mask(Discrete Event Inport){PermitSubsystemEvents=on, TypeOfEvent=Change in signal, SignalEdgeOption=Rising, SpecifyEventPriority=on, PrioritySubsystemEvent=600}
      mask prompts: PermitSubsystemEvents "Execute subsystem upon signal-based events"; TypeOfEvent "Type of signal-based event:"; SignalEdgeOption "Type of change in signal value:"; SpecifyEventPriority "Resolve simultaneous signal updates according to event priority"; PrioritySubsystemEvent "Event priority:"
      mask help: Input port for a Discrete Event Subsystem block. This block can conditionally execute the subsystem upon signal-based events that meet specified criteria.
      mask init:
      | des_subsystemmask(gcb, 'init','apply')
      settings: CopyFcn=des_subsysteminport(gcb, 'copy');  DeleteFcn=des_subsysteminport(gcb, 'delete');  UndoDeleteFcn=des_subsysteminport(gcb, 'undodelete');  ModelCloseFcn=des_subsysteminport(gcb, 'modelclose');  PreSaveFcn=des_subsysteminport(gcb, 'presave');  NameChangeFcn=des_subsysteminport(gcb, 'namechange');  ParentCloseFcn=des_subsysteminport(gcb, 'parentclose');
      mask Help: helpview(simeventsbhelp);
      mask StyleString: checkbox,popup(Change in signal|Trigger|Sample time hit),popup(Rising|Falling|Either),checkbox,edit
      mask CallbackString: des_subsystemmask(gcb, 'cbPermitSubsystemEvents', 'noapply');|des_subsystemmask(gcb,'cbTypeOfEvent','noapply');||des_subsystemmask(gcb, 'cbSpecifyEventPriority', 'noapply');|
  Subsystem Configuration : TriggerPort  TriggerType=function-call
      settings: CopyFcn=des_subsystemconfigblock(gcb, 'copy');  DeleteFcn=des_subsystemconfigblock(gcb, 'delete');  UndoDeleteFcn=des_subsystemconfigblock(gcb, 'undodelete');
      mask Type: Subsystem Configuration
      mask Description: Configuration for a Discrete Event Subsystem block. Every discrete event subsystem window must contain exactly one copy of this configuration block. Do not delete this block.
      mask Help: helpview(simeventsbhelp);
      mask Display: disp('Do Not Delete');
  Data Store Read : DataStoreRead  DataStoreName=n  SampleTime=-1
  Data Store Write : DataStoreWrite  DataStoreName=n  SampleTime=-1
  Embedded MATLAB Function : Stateflow chart  TreatAsAtomicUnit=on
  Unit Delay : UnitDelay  SampleTime=-1
  Unit Delay1 : UnitDelay  SampleTime=-1
  en : Outport  LoadFcn=des_subsystemoutport(gcb, 'load');  InitFcn=des_subsystemoutport(gcb, 'init');  StartFcn=des_subsystemoutport(gcb, 'start');  StopFcn=des_subsystemoutport(gcb, 'stop');  OutDataType=sfix(16)  OutScaling=2^0
      settings: CopyFcn=des_subsystemoutport(gcb, 'copy');  DeleteFcn=des_subsystemoutport(gcb, 'delete');  UndoDeleteFcn=des_subsystemoutport(gcb, 'undodelete');  ModelCloseFcn=des_subsystemoutport(gcb, 'modelclose');  PreSaveFcn=des_subsystemoutport(gcb, 'presave');  NameChangeFcn=des_subsystemoutport(gcb, 'namechange');  ParentCloseFcn=des_subsystemoutport(gcb, 'parentclose');
      mask Type: Discrete Event Outport
      mask Description: Provide an output port for a Discrete Event Subsystem block.
      mask Help: helpview(simeventsbhelp);
  wires:
  Unit Delay/1 -> Embedded MATLAB Function/5(en_in)
  Embedded MATLAB Function/1(en_out) -> Unit Delay/1, en/1
  Embedded MATLAB Function/2(n_out) -> Data Store Write/1
  Data Store Read/1 -> Embedded MATLAB Function/4(n_in)
  #n/1 -> Embedded MATLAB Function/1(state)
  #to/1 -> Embedded MATLAB Function/2(to), Unit Delay1/1
  Unit Delay1/1 -> Embedded MATLAB Function/3(old_to)

== matlab function Rate-Based Shared Processor/Scheduler/Scheduler for Task Arrival/Task Rescheudling Control/__fcn_ss__/Embedded MATLAB Function ==
  data: state input double; en_out output double; pe input double; n_in input double; en_in input double; n_out output double
function [en_out,n_out] = fcn(state,pe,n_in, en_in)
% This block supports the Embedded MATLAB subset.
% See the help menu for details. 

if (pe > n_in)
    n_out = n_in + 1;
    en_out = 1;
else
    if (state == n_in)
        n_out = n_in;
        en_out = 0;
    else
        n_out = n_in;
        en_out = en_in;
    end
end

== matlab function Rate-Based Shared Processor/Scheduler/Scheduler for Task Departure/Recompute Processing Time/Embedded MATLAB Function ==
  data: work_in input double; work_out output double; et input double; n input double; time_out output double
function [work_out,time_out] = fcn(work_in,et,n)

work_out = work_in - et/(n+1);
time_out = work_out * n;

== matlab function Rate-Based Shared Processor/Scheduler/Scheduler for Task Departure/Task Rescheduling Control/__fcn_ss__/Embedded MATLAB Function ==
  data: state input double; en_out output double; to input double; old_to input double; n_in input double; en_in input double; n_out output double
function [en_out,n_out] = fcn(state,to,old_to,n_in, en_in)
% This block supports the Embedded MATLAB subset.
% See the help menu for details. 

if (to > old_to)
    n_out = n_in - 1;
    en_out = 1;
else
    if (state == n_in)
        n_out = n_in;
        en_out = 0;
    elseif (state > n_in && en_in == 1)
        n_out = n_in;
        en_out = 0;
    else
        n_out = n_in;
        en_out = en_in;
    end
end

== matlab function Rate-Based Shared Processor/Scheduler/Scheduler for Task Arrival/Recompute Processing Time/Embedded MATLAB Function ==
  data: work_in input double; work_out output double; et input double; n input double; time_out output double
function [work_out,time_out] = fcn(work_in,et,n)

if n==1
    work_out = work_in;
    time_out = work_in;
else
    work_out = work_in - et/(n-1);
    time_out = work_out * n;
end

== matlab function Rate-Based Shared Processor/Task Admission Control/__fcn_ss__/Embedded MATLAB Function ==
  data: to input double; to_old input double; en_out output double; pe input double; n_in input double; en_in input double; state input double
function en_out = fcn(to,to_old,pe,n_in,en_in,state)
% This block supports the Embedded MATLAB subset.
% See the help menu for details. 

if (to > to_old)
    en_out = 0;
else
    if (pe == n_in && state > 0)
        en_out = 1;
    elseif (pe > n_in)
        en_out = 0;
    else
        en_out = en_in;
    end
end
